simulink model "Coil"  (R2021b)
settings: Solver=FixedStepAuto  StartTime=-6000e-6  StopTime=6000e-6  FixedStep=25e-6  RelTol=1e-3
libraries: simulink x1
(part 2 of 2)

== matlab function Coil/Outer_5_Coils/Square-7/Square - 7 ==
  data: x input; F_xx_7 output; F_xz_7 output; y input; z input; I input; F_yy_7 output; F_yz_7 output
function [F_xx_7, F_xz_7, F_yy_7, F_yz_7] = force(x, y, z, I)

g = 417.14e-6;     %Coil spacing
m0 = 4*pi*1e-7;
radius = 3e-3;%m
height = 1e-3;%m
Magentization = 1.45; %T
vol_cy = pi*radius^2*height; %If Object is Cylinder, vol in m^3
% vol_sp = (4/3)*(pi * radius^3); %If Object is Sphere, vol in m^3

k = 0.4e-3; %additional length added to wires, to get concentric coil
%--------%--------%--------%--------%--------%--------%--------%----------
% Line along y - axis
%-%--------%--------%--------%--------%--------%--------%--------%--------
yp1_1 = -0.6e-3 - 6*k;
yp2_1 = 0.6e-3 + 6*k;
yn1_1 = -0.8e-3 - 6*k;
yn2_1 = 0.8e-3 + 6*k;
a_xp_1 = 7*g;  
a_xn_1 = -7*g;

k_yp_1 = 1/(4*pi*((a_xp_1-x)^2+z^2));
k_1yp_1 = (yp2_1-y)/((yp2_1-y)^2+(a_xp_1-x)^2+z^2)^0.5;
k_2yp_1 = (yp1_1-y)/((yp1_1-y)^2+(a_xp_1-x)^2+z^2)^0.5;

k_1yp_3 = (yp2_1-y)/((yp2_1-y)^2+(a_xp_1-x)^2+z^2)^1.5;
k_2yp_3 = (yp1_1-y)/((yp1_1-y)^2+(a_xp_1-x)^2+z^2)^1.5;

k_yn_1 = 1/(4*pi*((a_xn_1-x)^2+z^2));
k_1yn_1 = (yn2_1-y)/((yn2_1-y)^2+(a_xn_1-x)^2+z^2)^0.5;
k_2yn_1 = (yn1_1-y)/((yn1_1-y)^2+(a_xn_1-x)^2+z^2)^0.5;

k_1yn_3 = (yn2_1-y)/((yn2_1-y)^2+(a_xn_1-x)^2+z^2)^1.5;
k_2yn_3 = (yn1_1-y)/((yn1_1-y)^2+(a_xn_1-x)^2+z^2)^1.5;

hyp_x_1 = -(z*k_yp_1*(a_xp_1-x))*I*m0;
hyp_x1_1 = (k_yp_1*(k_1yp_1 - k_2yp_1))*2*4*pi;
hyp_x2_1 = k_1yp_3 - k_2yp_3;
dBxp_1_dx = hyp_x_1*(hyp_x1_1 + hyp_x2_1);

hyp_z_1 = (k_yp_1)*I*m0;
hyp_z1_1 = (k_1yp_1 - k_2yp_1)*(-1);
hyp_z2_1 = (k_yp_1*(k_1yp_1 - k_2yp_1)*(z^2))*4*pi*2;
hyp_z3_1 = (k_1yp_3 - k_2yp_3)*(z^2);
dBxp_1_dz = hyp_z_1*(hyp_z1_1 + hyp_z2_1 + hyp_z3_1);

hyn_x_1 = -(z*k_yn_1*(a_xn_1-x))*I*m0*(-1);
hyn_x1_1 = (k_yn_1*(k_1yn_1 - k_2yn_1))*2*4*pi;
hyn_x2_1 = k_1yn_3 - k_2yn_3;
dBxn_1_dx = hyn_x_1*(hyn_x1_1 + hyn_x2_1);

hyn_z_1 = (k_yn_1)*I*m0*(-1);
hyn_z1_1 = (k_1yn_1 - k_2yn_1)*(-1);
hyn_z2_1 = (k_yn_1*(k_1yn_1 - k_2yn_1)*(z^2))*4*pi*2;
hyn_z3_1 = (k_1yn_3 - k_2yn_3)*(z^2);
dBxn_1_dz = hyn_z_1*(hyn_z1_1 + hyn_z2_1 + hyn_z3_1);

%--------%--------%--------%--------%--------%--------%--------%----------
% Line along x - axis
%-%--------%--------%--------%--------%a--------%--------%--------%--------
xp1_1 = -0.8e-3 - 6*k;
xp2_1 = 0.8e-3 + 6*k;
xn1_1 = -1e-3 - 6*k;
xn2_1 = 1e-3 + 6*k;
a_yp_1 = 3.075e-3;          %Distance of coil from (0,0)
a_yn_1 = -3.075e-3;

k_xp_1 = 1/(4*pi*((a_yp_1-y)^2+z^2));
k_1xp_1 = (xp2_1-x)/((xp2_1-x)^2+(a_yp_1-y)^2+z^2)^0.5;
k_2xp_1 = (xp1_1-x)/((xp1_1-x)^2+(a_yp_1-y)^2+z^2)^0.5;

k_xn_1 = 1/(4*pi*((a_yn_1-y)^2+z^2));
k_1xn_1 = (xn2_1-x)/((xn2_1-x)^2+(a_yn_1-y)^2+z^2)^0.5;
k_2xn_1 = (xn1_1-x)/((xn1_1-x)^2+(a_yn_1-y)^2+z^2)^0.5;

k_1xp_3 = (xp2_1-x)/((xp2_1-x)^2+(a_yp_1-y)^2+z^2)^1.5;
k_2xp_3 = (xp1_1-x)/((xp1_1-x)^2+(a_yp_1-y)^2+z^2)^1.5;

k_1xn_3 = (xn2_1-x)/((xn2_1-x)^2+(a_yn_1-y)^2+z^2)^1.5;
k_2xn_3 = (xn1_1-x)/((xn1_1-x)^2+(a_yn_1-y)^2+z^2)^1.5;

hxp_x_1 = -(z*k_xp_1*(a_yp_1-y))*I*m0;
hxp_x1_1 = (k_xp_1*(k_1xp_1 - k_2xp_1))*2*4*pi;
hxp_x2_1 = k_1xp_3 - k_2xp_3;
dByp_1_dy = hxp_x_1*(hxp_x1_1 + hxp_x2_1);

hxp_z_1 = (k_xp_1)*I*m0;
hxp_z1_1 = (k_1xp_1 - k_2xp_1)*(-1);
hxp_z2_1 = (k_xp_1*(k_1xp_1 - k_2xp_1)*(z^2))*4*pi*2;
hxp_z3_1 = (k_1xp_3 - k_2xp_3)*(z^2);
dByp_1_dz = hxp_z_1*(hxp_z1_1 + hxp_z2_1 + hxp_z3_1);

hxn_x_1 = -(z*k_xn_1*(a_yn_1-y))*I*m0*(-1);
hxn_x1_1 = (k_xn_1*(k_1xn_1 - k_2xn_1))*2*4*pi;
hxn_x2_1 = k_1xn_3 - k_2xn_3;
dByn_1_dy = hxn_x_1*(hxn_x1_1 + hxn_x2_1);

hxn_z_1 = (k_xn_1)*I*m0*(-1);
hxn_z1_1 = (k_1xn_1 - k_2xn_1)*(-1);
hxn_z2_1 = (k_xn_1*(k_1xn_1 - k_2xn_1)*(z^2))*4*pi*2;
hxn_z3_1 = (k_1xn_3 - k_2xn_3)*(z^2);
dByn_1_dz = hxn_z_1*(hxn_z1_1 + hxn_z2_1 + hxn_z3_1);

F_xx_7 = vol_cy * Magentization* (dBxp_1_dx + dBxn_1_dx)/m0;
F_xz_7 = vol_cy * Magentization* (dBxp_1_dz + dBxn_1_dz)/m0;
F_yy_7 = vol_cy * Magentization* (dByp_1_dy + dByn_1_dy)/m0;
F_yz_7 = vol_cy * Magentization* (dByp_1_dz + dByn_1_dz)/m0;
end
